simulink model "BMS_Software"  (R2022b)
settings: configuration reference "BMS_Sw_CodeGenConfig" (kept outside this file)
undefined symbols (not defined in the file or in its folder): ts
settings Model: DataDictionary=Shared_DD.sldd  EnableAccessToBaseWorkspace=off  PauseTimes=0  ExtModeTrigDuration=5  Creator=Chirag Patel  LastModifiedBy=salem
settings ConfigSetRef: SourceName=BMS_Sw_CodeGenConfig

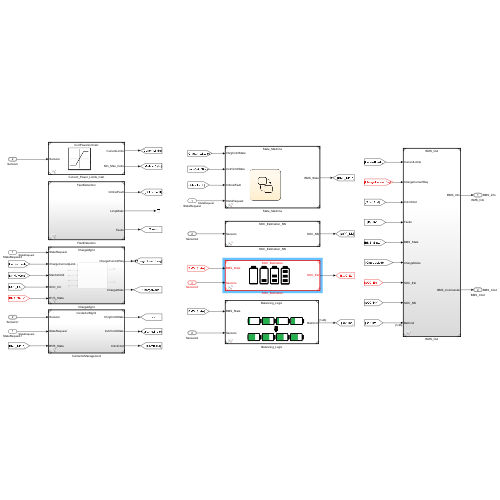
[thumbnail: Simulink's stored preview of the top-level diagram]
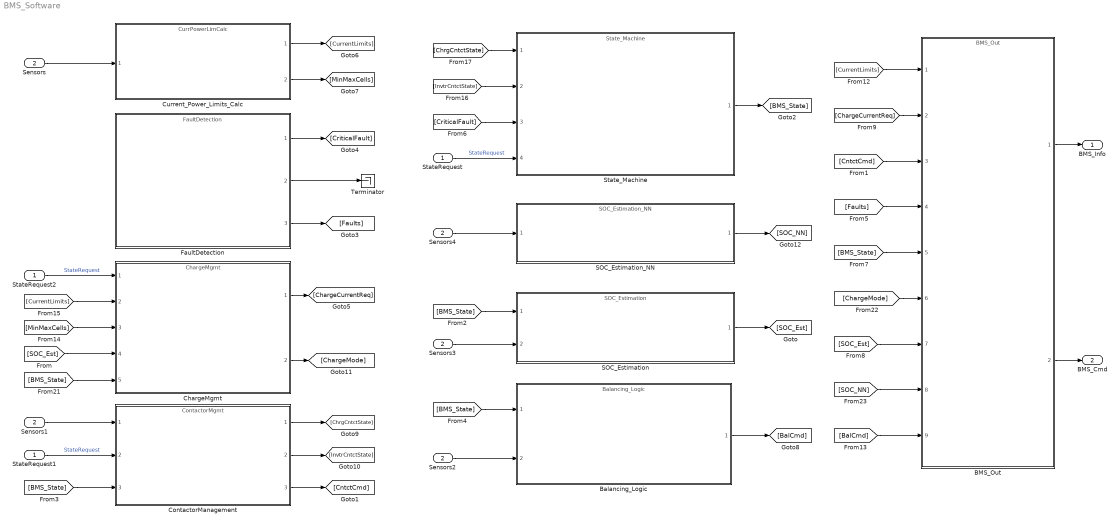
== system BMS_Software ==
  StateRequest : Inport  OutDataTypeStr=Enum: SRE  PortDimensions=1  SampleTime=ts
  Sensors : Inport  Port=2  OutDataTypeStr=Bus: Sensors  BusOutputAsStruct=on
  BMS_Out : ModelReference  ModelNameDialog=BMS_Out.slx  SimulationMode=Normal  ModelReferenceVersion=5.2
  Balancing_Logic : ModelReference  ModelNameDialog=Balancing_Logic  SimulationMode=Normal  ModelReferenceVersion=5.19
      mask Display: image('Balancing.jpg',[75,5,200,90])
  ChargeMgmt : ModelReference  ModelNameDialog=ChargeMgmt.slx  SimulationMode=Normal  ModelReferenceVersion=2.14
  ContactorManagement : ModelReference  ModelNameDialog=ContactorMgmt.slx  SimulationMode=Normal  ModelReferenceVersion=5.16
  Current_Power_Limits_Calc : ModelReference  ModelNameDialog=CurrPowerLimCalc.slx  SimulationMode=Normal  ModelReferenceVersion=5.32
      mask Display: image('CurrentPowerLimit.png',[68,15,80,80])
  FaultDetection : ModelReference  ModelNameDialog=FaultDetection  SimulationMode=Normal  ModelReferenceVersion=5.26
  SOC_Estimation : ModelReference  ModelNameDialog=SOC_Estimation.slx  SimulationMode=Normal  ModelReferenceVersion=5.40
      mask Display: image('SOC.jpg',[80,15,150,75])
  SOC_Estimation_NN : ModelReference  ModelNameDialog=SOC_Estimation_NN.slx  SimulationMode=Normal  ModelReferenceVersion=5.34
  Sensors{1..4} (4 alike) : InportShadow  Port=2  OutDataTypeStr=Bus: Sensors  BusOutputAsStruct=on
  StateRequest1 : InportShadow  OutDataTypeStr=Enum: SRE  PortDimensions=1  SampleTime=ts
  StateRequest2 : InportShadow  OutDataTypeStr=Enum: SRE  PortDimensions=1  SampleTime=ts
  State_Machine : ModelReference  ModelNameDialog=State_Machine  SimulationMode=Normal  ModelReferenceVersion=5.4
      mask Display: image('StateMachine.jpg',[80,20,120,120])
  Terminator : Terminator
  BMS_Info : Outport  SignalName=BMS_Info  OutDataTypeStr=Bus: BMS_Info  VectorParamsAs1DForOutWhenUnconnected=off  BusOutputAsStruct=on
  BMS_Cmd : Outport  Port=2  SignalName=BMS_Cmd  OutDataTypeStr=Bus: BMS_Cmd  VectorParamsAs1DForOutWhenUnconnected=off  BusOutputAsStruct=on
  wires:
  Sensors3/1 -> SOC_Estimation/2
  SOC_Estimation/1 -> [SOC_Est]
  Sensors2/1 -> Balancing_Logic/2
  [BMS_State] -> Balancing_Logic/1
  StateRequest1/1 -> ContactorManagement/2  "StateRequest"
  [BMS_State] -> ContactorManagement/3
  [CntctCmd] -> BMS_Out/3
  [BMS_State] -> SOC_Estimation/1
  BMS_Out/1 -> BMS_Info/1
  BMS_Out/2 -> BMS_Cmd/1
  Sensors/1 -> Current_Power_Limits_Calc/1
  State_Machine/1 -> [BMS_State]
  [Faults] -> BMS_Out/4
  ContactorManagement/3 -> [CntctCmd]
  StateRequest/1 -> State_Machine/4  "StateRequest"
  [BMS_State] -> BMS_Out/5
  [ChargeCurrentReq] -> BMS_Out/2
  Current_Power_Limits_Calc/1 -> [CurrentLimits]
  Current_Power_Limits_Calc/2 -> [MinMaxCells]
  [CurrentLimits] -> BMS_Out/1
  Balancing_Logic/1 -> [BalCmd]
  ContactorManagement/1 -> [ChrgCntctState]
  ContactorManagement/2 -> [InvtrCntctState]
  [MinMaxCells] -> ChargeMgmt/3
  [CurrentLimits] -> ChargeMgmt/2
  StateRequest2/1 -> ChargeMgmt/1  "StateRequest"
  Sensors1/1 -> ContactorManagement/1
  [SOC_Est] -> ChargeMgmt/4
  [ChrgCntctState] -> State_Machine/1
  [InvtrCntctState] -> State_Machine/2
  [CriticalFault] -> State_Machine/3
  ChargeMgmt/1 -> [ChargeCurrentReq]
  ChargeMgmt/2 -> [ChargeMode]
  [BMS_State] -> ChargeMgmt/5
  [ChargeMode] -> BMS_Out/6
  [BalCmd] -> BMS_Out/9
  [SOC_Est] -> BMS_Out/7
  Sensors4/1 -> SOC_Estimation_NN/1
  SOC_Estimation_NN/1 -> [SOC_NN]
  [SOC_NN] -> BMS_Out/8
  FaultDetection/1 -> [CriticalFault]
  FaultDetection/3 -> [Faults]
  FaultDetection/2 -> Terminator/1
